simulink library "SyDdemoChildren"  (Simulink 7.0)
undefined symbols (not defined in the file): BATTERY_COR_ENA, BATTERY_COR_PWM, DIAG_AIR_ESTI_ERROR_MAX, DIAG_ATMO_PRESSURE_MAX, DIAG_COOLANT_TEMP_MAX, DIAG_COOLANT_TEMP_MIN, DIAG_ENGINE_SPEED_MAX, DIAG_ENGINE_SPEED_MIN, DIAG_POS_DMND_RAW_MIN, RUNNING
libraries: simulink x3
settings Model: Creator=LeanPulse  LastModifiedBy=LeanPulse
settings Model: ModifiedHistory=|
  | <syd:extradata xmlns:syd="http://www.leanpulse.com/schemas/syd/2011/core" owner="LeanPulse" ref="SPEC0002" title="SyD Demo - Children Systems"><syd:version author="Aurélien PROST" date="15 October 2014" num="1.0" opt1="" opt2="">This model is referenced by the root demo model "SyDdemo.mdl". It has been created to highlight the generation of multiple documents by following the model links, as enabled by SyD.
  | 
  | (c) LeanPulse 2014</syd:version></syd:extradata>

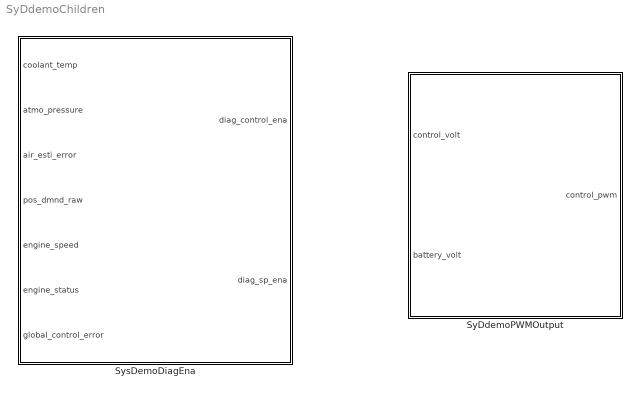
== system SyDdemoChildren ==
  SyDdemoPWMOutput : Subsystem
  SysDemoDiagEna : Subsystem

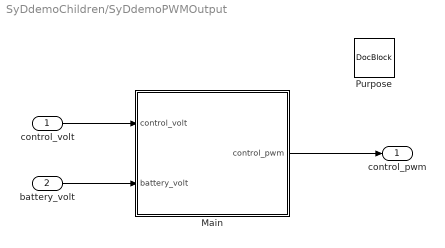
== system SyDdemoChildren/SyDdemoPWMOutput ==
  control_volt : Inport
  battery_volt : Inport  Port=2
  Main : Subsystem
  Purpose : simulink/Model-Wide Utilities/DocBlock  SystemSampleTime=-1  DocumentType=RTF
  control_pwm : Outport
  wires:
  control_volt/1 -> Main/1(control_volt)
  battery_volt/1 -> Main/2(battery_volt)
  Main/1(control_pwm) -> control_pwm/1

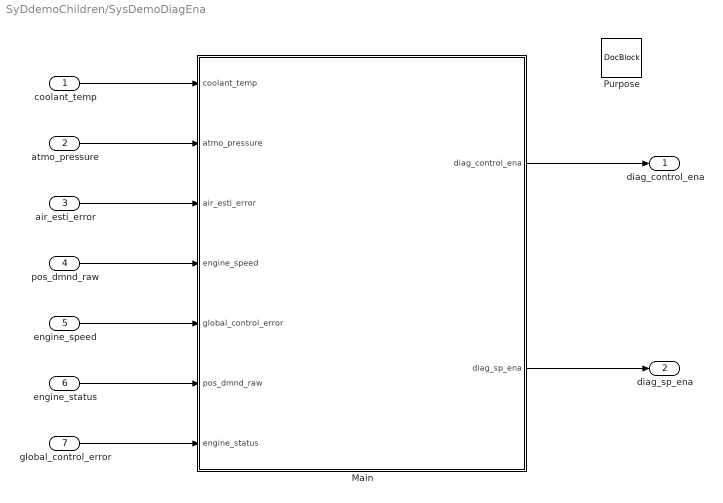
== system SyDdemoChildren/SysDemoDiagEna ==
  coolant_temp : Inport
  atmo_pressure : Inport  Port=2
  air_esti_error : Inport  Port=3
  pos_dmnd_raw : Inport  Port=4
  engine_speed : Inport  Port=5
  engine_status : Inport  Port=6
  global_control_error : Inport  Port=7
  Main : Subsystem
  Purpose : simulink/Model-Wide Utilities/DocBlock  SystemSampleTime=-1  DocumentType=RTF
  diag_control_ena : Outport
  diag_sp_ena : Outport  Port=2
  wires:
  Main/1(diag_control_ena) -> diag_control_ena/1
  Main/2(diag_sp_ena) -> diag_sp_ena/1
  coolant_temp/1 -> Main/1(coolant_temp)
  atmo_pressure/1 -> Main/2(atmo_pressure)
  air_esti_error/1 -> Main/3(air_esti_error)
  pos_dmnd_raw/1 -> Main/4(engine_speed)
  engine_speed/1 -> Main/5(global_control_error)
  engine_status/1 -> Main/6(pos_dmnd_raw)
  global_control_error/1 -> Main/7(engine_status)

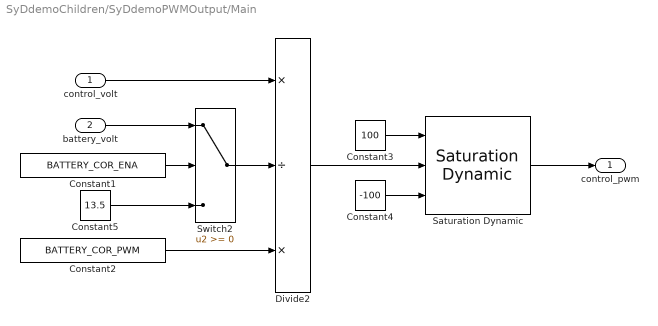
== system SyDdemoChildren/SyDdemoPWMOutput/Main ==
  control_volt : Inport
  battery_volt : Inport  Port=2
  Constant1 : Constant  Value=BATTERY_COR_ENA
  Constant2 : Constant  Value=BATTERY_COR_PWM
  Constant3 : Constant  Value=100
  Constant4 : Constant  Value=-100
  Constant5 : Constant  Value=13.5
  Divide2 : Product  Inputs=*/*
  Saturation Dynamic : simulink/Discontinuities/Saturation Dynamic  SystemSampleTime=-1  OutMin=[]  OutMax=[]  OutDataType=fixdt(1, 16)  OutScaling=2^-10  DoSatur=off
  Switch2 : Switch
  control_pwm : Outport
  wires:
  battery_volt/1 -> Switch2/1
  Constant1/1 -> Switch2/2
  Constant5/1 -> Switch2/3
  Switch2/1 -> Divide2/2
  control_volt/1 -> Divide2/1
  Constant2/1 -> Divide2/3
  Divide2/1 -> Saturation Dynamic/2
  Constant4/1 -> Saturation Dynamic/3
  Constant3/1 -> Saturation Dynamic/1
  Saturation Dynamic/1 -> control_pwm/1

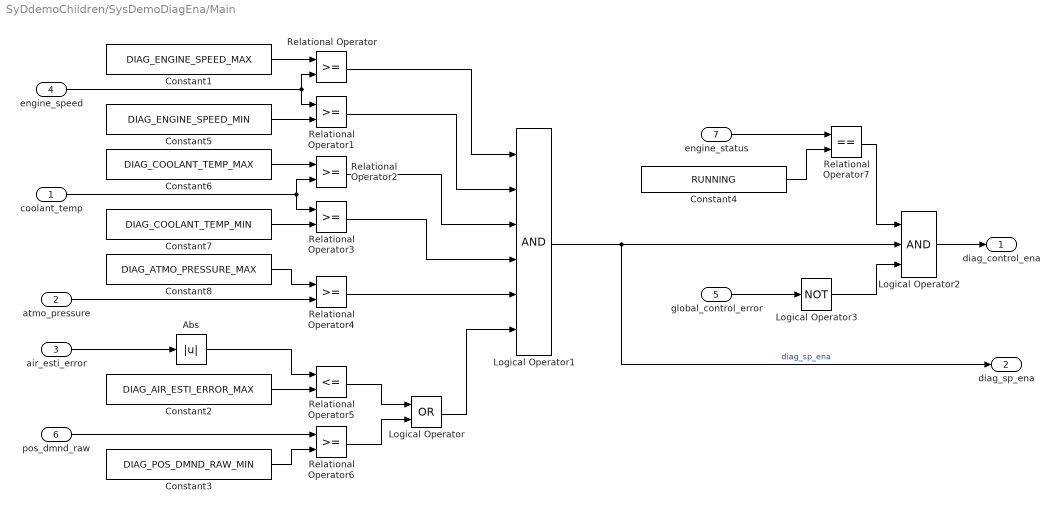
== system SyDdemoChildren/SysDemoDiagEna/Main ==
  coolant_temp : Inport
  atmo_pressure : Inport  Port=2
  air_esti_error : Inport  Port=3
  engine_speed : Inport  Port=4
  global_control_error : Inport  Port=5
  pos_dmnd_raw : Inport  Port=6
  engine_status : Inport  Port=7
  Abs : Abs
  Constant1 : Constant  Value=DIAG_ENGINE_SPEED_MAX
  Constant2 : Constant  Value=DIAG_AIR_ESTI_ERROR_MAX
  Constant3 : Constant  Value=DIAG_POS_DMND_RAW_MIN
  Constant4 : Constant  Value=RUNNING
  Constant5 : Constant  Value=DIAG_ENGINE_SPEED_MIN
  Constant6 : Constant  Value=DIAG_COOLANT_TEMP_MAX
  Constant7 : Constant  Value=DIAG_COOLANT_TEMP_MIN
  Constant8 : Constant  Value=DIAG_ATMO_PRESSURE_MAX
  Logical Operator : Logic  Operator=OR  AllPortsSameDT=off  OutDataTypeMode=boolean
  Logical Operator1 : Logic  Inputs=6  AllPortsSameDT=off  OutDataTypeMode=boolean
  Logical Operator2 : Logic  Inputs=3  AllPortsSameDT=off  OutDataTypeMode=boolean
  Logical Operator3 : Logic  Operator=NOT  AllPortsSameDT=off  OutDataTypeMode=boolean
  Relational Operator{,1..4,6} (6 alike) : RelationalOperator  LogicOutDataTypeMode=boolean
  Relational Operator5 : RelationalOperator  Operator=<=  LogicOutDataTypeMode=boolean
  Relational Operator7 : RelationalOperator  Operator===  LogicOutDataTypeMode=boolean
  diag_control_ena : Outport
  diag_sp_ena : Outport  Port=2
  wires:
  engine_speed/1 -> Relational Operator/2, Relational Operator1/1
  Constant1/1 -> Relational Operator/1
  Constant5/1 -> Relational Operator1/2
  coolant_temp/1 -> Relational Operator2/2, Relational Operator3/1
  Constant6/1 -> Relational Operator2/1
  Constant7/1 -> Relational Operator3/2
  atmo_pressure/1 -> Relational Operator4/2
  Constant8/1 -> Relational Operator4/1
  air_esti_error/1 -> Abs/1
  Abs/1 -> Relational Operator5/1
  Constant2/1 -> Relational Operator5/2
  pos_dmnd_raw/1 -> Relational Operator6/1
  Constant3/1 -> Relational Operator6/2
  Relational Operator5/1 -> Logical Operator/1
  Relational Operator6/1 -> Logical Operator/2
  Relational Operator/1 -> Logical Operator1/1
  Relational Operator1/1 -> Logical Operator1/2
  Relational Operator2/1 -> Logical Operator1/3
  Relational Operator3/1 -> Logical Operator1/4
  Relational Operator4/1 -> Logical Operator1/5
  Logical Operator/1 -> Logical Operator1/6
  Logical Operator1/1 -> Logical Operator2/2, diag_sp_ena/1  "diag_sp_ena"
  Constant4/1 -> Relational Operator7/2
  engine_status/1 -> Relational Operator7/1
  Relational Operator7/1 -> Logical Operator2/1
  global_control_error/1 -> Logical Operator3/1
  Logical Operator3/1 -> Logical Operator2/3
  Logical Operator2/1 -> diag_control_ena/1
